simulink model "2 - Damper Problem"  (R2020b)
settings: Solver=VariableStepAuto  StartTime=0.0  StopTime=20  RelTol=1e-3
settings Model: Creator=hooshmand  LastModifiedBy=hooshmand

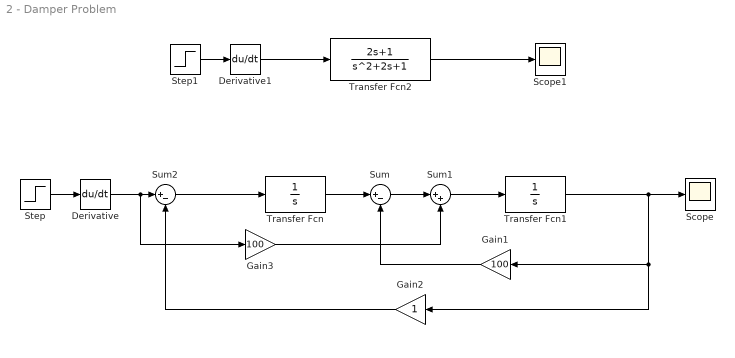
== system 2 - Damper Problem ==
  Derivative : Derivative
  Derivative1 : Derivative
  Gain1 : Gain  Gain=100
  Gain2 : Gain
  Gain3 : Gain  Gain=100
  Scope : Scope
  Scope1 : Scope
  Step : Step  Time=0.001  SampleTime=0
  Step1 : Step  Time=10  SampleTime=0
  Sum : Sum  Inputs=|+-
  Sum1 : Sum  Inputs=|++
  Sum2 : Sum  Inputs=|+-
  Transfer Fcn : TransferFcn  Denominator=[1 0]
  Transfer Fcn1 : TransferFcn  Denominator=[1 0]
  Transfer Fcn2 : TransferFcn  Numerator=[2 1]
  wires:
  Step/1 -> Derivative/1
  Transfer Fcn1/1 -> Gain1/1, Gain2/1, Scope/1
  Sum1/1 -> Transfer Fcn1/1
  Sum/1 -> Sum1/1
  Transfer Fcn/1 -> Sum/1
  Gain2/1 -> Sum2/2
  Gain1/1 -> Sum/2
  Sum2/1 -> Transfer Fcn/1
  Gain3/1 -> Sum1/2
  Derivative/1 -> Gain3/1, Sum2/1
  Step1/1 -> Derivative1/1
  Derivative1/1 -> Transfer Fcn2/1
  Transfer Fcn2/1 -> Scope1/1
